simulink library "lib_configurable_parameter"  (R2023a)
settings: Solver=VariableStepAuto  StartTime=0.0  StopTime=10.0  RelTol=1e-3
settings Model: Creator=cav2ofo  LastModifiedBy=lenovo
settings OptimizationCC: ReuseModelBlockBuffer=off

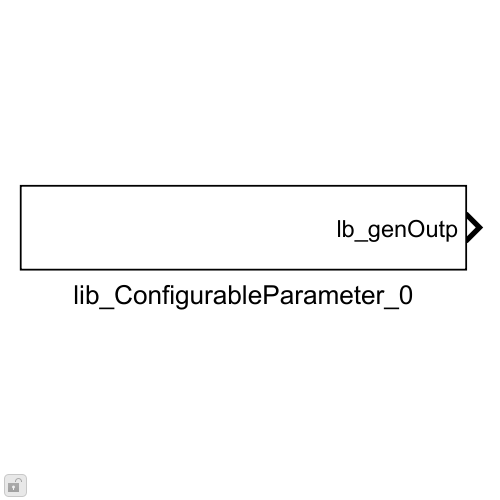
[thumbnail: Simulink's stored preview of the top-level diagram]
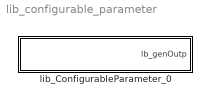
== system lib_configurable_parameter ==
  lib_ConfigurableParameter_0 : Subsystem  mask{lb_parCnfgPar=1, lb_parDataType=Inherit: Inherit from 'Constant value', lb_parUpLim=2, lb_parLowLim=0}
      mask prompts: lb_parCnfgPar "Configurable parameter:"; lb_parDataType "Simulink:blkprm_prompts:OUTPUT_UNIFIEDDATATYPE"; lb_parUpLim "Simulink:blkprm_prompts:SaturateUpLim"; lb_parLowLim "Simulink:blkprm_prompts:SaturateLowLim"
      mask init:
      | if lb_parUpLim == lb_parLowLim
      |     set_param([gcb,'/vss_SaturationActivation'],'LabelModeActiveChoice','lb_parSatNotReqLbl');
      | else
      |     set_param([gcb,'/vss_SaturationActivation'],'LabelModeActiveChoice','lb_parSatReqLbl');
      | end
      mask TypeOptions lb_parCnfgPar: vss_SaturationActivation/vss_SaturationRequired/Constant/Value | vss_SaturationActivation/vss_SaturationNotRequired/Constant/Value
      mask TypeOptions lb_parDataType: vss_SaturationActivation/vss_SaturationNotRequired/Constant/OutDataTypeStr | vss_SaturationActivation/vss_SaturationRequired/Constant/OutDataTypeStr
      mask TypeOptions lb_parUpLim: vss_SaturationActivation/vss_SaturationRequired/Saturation/UpperLimit
      mask TypeOptions lb_parLowLim: vss_SaturationActivation/vss_SaturationRequired/Saturation/LowerLimit
      mask DialogControl DescGroupVar Prompt: VHIT control library
      mask DialogControl DescTextVar Prompt: Data type conversion and duplicate
      mask DialogControl lb_parDataType Prompt: 输出数据类型:
      mask DialogControl lb_parUpLim Prompt: 上限:
      mask DialogControl lb_parLowLim Prompt: 下限:

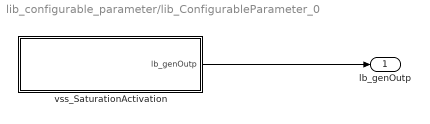
== system lib_configurable_parameter/lib_ConfigurableParameter_0 ==
  vss_SaturationActivation : Subsystem  Variant=on  VariantControlMode=label  LabelModeActiveChoice=lb_parSatReqLbl
  lb_genOutp : Outport
  wires:
  vss_SaturationActivation/1(lb_genOutp) -> lb_genOutp/1

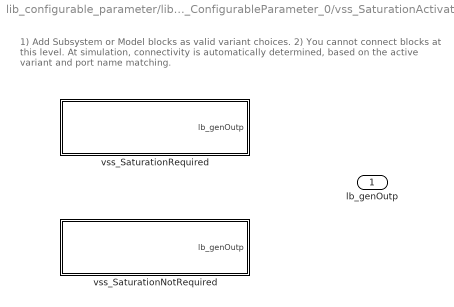
== system lib_configurable_parameter/lib_ConfigurableParameter_0/vss_SaturationActivation ==
  note: 1) Add Subsystem or Model blocks as valid variant choices.
      | 2) You cannot connect blocks at this level. At simulation, connectivity is automatically
      | determined, based on the active variant and port name matching.
  vss_SaturationNotRequired : Subsystem  VariantControl=lb_parSatNotReqLbl
  vss_SaturationRequired : Subsystem  VariantControl=lb_parSatReqLbl
  lb_genOutp : Outport

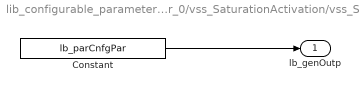
== system lib_configurable_parameter/lib_ConfigurableParameter_0/vss_SaturationActivation/vss_SaturationNotRequired ==
  Constant : Constant  Value=lb_parCnfgPar
  lb_genOutp : Outport
  wires:
  Constant/1 -> lb_genOutp/1

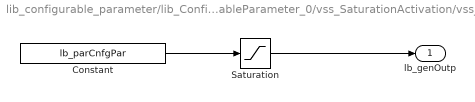
== system lib_configurable_parameter/lib_ConfigurableParameter_0/vss_SaturationActivation/vss_SaturationRequired ==
  Constant : Constant  Value=lb_parCnfgPar
  Saturation : Saturate  UpperLimit=lb_parUpLim  LowerLimit=lb_parLowLim
  lb_genOutp : Outport
  wires:
  Constant/1 -> Saturation/1
  Saturation/1 -> lb_genOutp/1
